simulink model "ACC_SWC"  (R2022b)
settings: configuration reference "ACC_AutosarConfig" (kept outside this file)
model workspace (MATLAB code in the model file):
  | cmdLim = Simulink.Parameter;
  | cmdLim.Value = 15;
  | cmdLim.Description = 'Limit for controlling the maximum surface command angle.';
  | cmdLim.Min = 0;
  | cmdLim.Max = 90;
  | cmdLim.DocUnits = 'deg';
  | 
  | dispGain = Simulink.Parameter;
  | dispGain.Value = 0.75;
  | dispGain.Description = 'Gain applied to the displacement error.';
  | dispGain.Min = 0;
  | dispGain.Max = [];
  | dispGain.DocUnits = 'deg/sec/deg';
  | 
  | dispLim = Simulink.Parameter;
  | dispLim.Value = 30;
  | dispLim.Description = 'Limit for controlling the maximum commanded angle.';
  | dispLim.Min = 0;
  | dispLim.Max = 180;
  | dispLim.DocUnits = 'deg';
  | 
  | intGain = Simulink.Parameter;
  | intGain.Value = 0.5;
  | intGain.Description = 'Gain applied to the integral error.';
  | intGain.Min = 0;
  | intGain.Max = [];
  | intGain.DocUnits = 'deg/sec/deg/sec';
  | 
  | intLim = Simulink.Parameter;
  | intLim.Value = 5;
  | intLim.Description = 'Limit for controlling the maximum commanded angle.';
  | intLim.Min = 0;
  | intLim.Max = 90;
  | intLim.DocUnits = 'deg';
  | 
  | rateGain = Simulink.Parameter;
  | rateGain.Value = 2;
  | rateGain.Description = 'Gain applied to the rate error.';
  | rateGain.Min = 0;
  | rateGain.Max = [];
  | rateGain.DocUnits = 'deg/deg/sec';
  | 
  | rateLim = Simulink.Parameter;
  | rateLim.Value = 6;
  | rateLim.Description = 'Limit for controlling the maximum commanded angle.';
  | rateLim.Min = 0;
  | rateLim.Max = 180;
  | rateLim.DocUnits = 'deg/sec';
  | 
  | hdgGain = Simulink.Parameter;
  | hdgGain.Value = 0.015;
values from neighbouring files (symbols this model uses):
  ACC_SampleTime = 0.01    [ACC_DD.sldd]
  Dem_EventStatusType : value not decoded    [ACC_DD.sldd]
libraries: autosarlibnvm x3, autosarlibdem x1
settings Model: RequirementInfo={} %GIDa_fe9045fd_0412_4b6e_8206_617cc20e6fde  DataDictionary=ACC_DD.sldd  FPTRunName=Active  Creator=MAAM  LastModifiedBy=MAAM
settings ConfigSetRef: SourceName=ACC_AutosarConfig

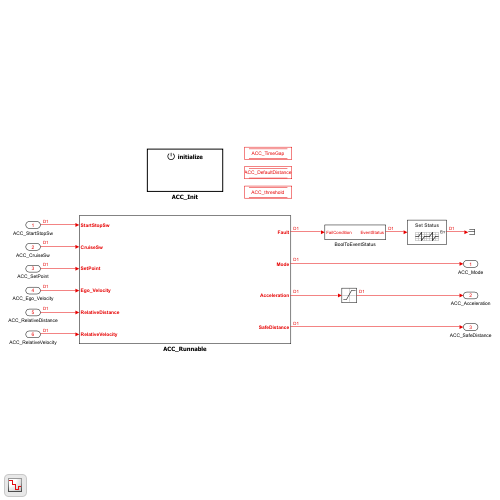
[thumbnail: Simulink's stored preview of the top-level diagram]
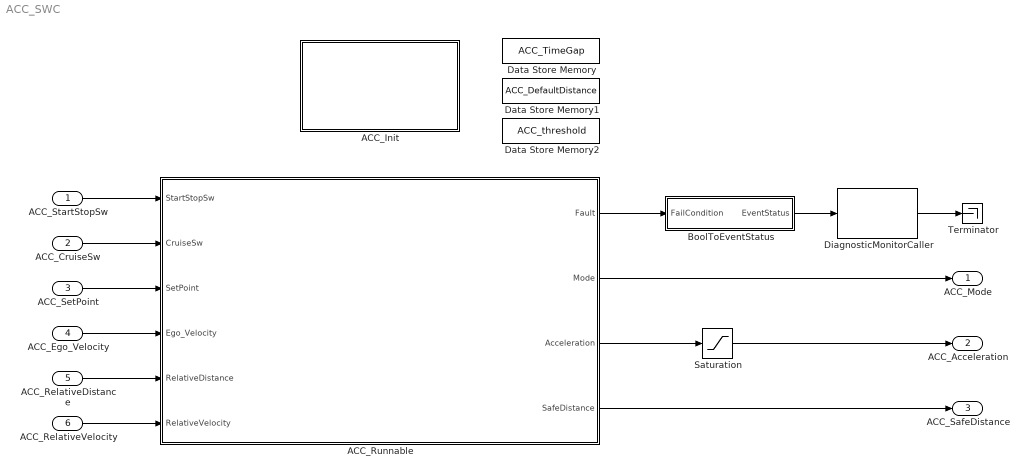
== system ACC_SWC ==
  ACC_StartStopSw : Inport  OutDataTypeStr=boolean  SampleTime=ACC_SampleTime
  ACC_CruiseSw : Inport  Port=2  OutDataTypeStr=boolean  SampleTime=ACC_SampleTime
  ACC_SetPoint : Inport  Port=3  OutDataTypeStr=single  SampleTime=ACC_SampleTime
  ACC_Ego_Velocity : Inport  Port=4  OutDataTypeStr=single  SampleTime=ACC_SampleTime
  ACC_RelativeDistance : Inport  Port=5  OutDataTypeStr=single  SampleTime=ACC_SampleTime
  ACC_RelativeVelocity : Inport  Port=6  OutDataTypeStr=single  SampleTime=ACC_SampleTime
  ACC_Init : Subsystem  TreatAsAtomicUnit=on
  ACC_Runnable : Subsystem  SystemSampleTime=1
  BoolToEventStatus : Subsystem
  Data Store Memory : DataStoreMemory  DataStoreName=ACC_TimeGap  WriteAfterWriteMsg=warning  ShowAdditionalParam=off  OutDataTypeStr=uint8
  Data Store Memory1 : DataStoreMemory  DataStoreName=ACC_DefaultDistance  WriteAfterWriteMsg=warning  ShowAdditionalParam=off  OutDataTypeStr=uint8
  Data Store Memory2 : DataStoreMemory  DataStoreName=ACC_threshold  WriteAfterWriteMsg=warning  ShowAdditionalParam=off  OutDataTypeStr=uint8
  DiagnosticMonitorCaller : autosarlibdem/DiagnosticMonitorCaller  PortName=ACC_Fail  Operation=SetEventStatus  Datatype=Enum: Dem_EventStatusType  st=-1  ServiceImpl=autosar.bsw.DemDiagnosticMonitor
  Saturation : Saturate  UpperLimit=10  LowerLimit=-10  OutDataTypeStr=single
  Terminator : Terminator
  ACC_Mode : Outport
  ACC_Acceleration : Outport  Port=2
  ACC_SafeDistance : Outport  Port=3
  wires:
  ACC_Runnable/4(SafeDistance) -> ACC_SafeDistance/1
  ACC_Runnable/3(Acceleration) -> Saturation/1
  ACC_Runnable/2(Mode) -> ACC_Mode/1
  ACC_Runnable/1(Fault) -> BoolToEventStatus/1(FailCondition)
  ACC_RelativeVelocity/1 -> ACC_Runnable/6(RelativeVelocity)
  ACC_RelativeDistance/1 -> ACC_Runnable/5(RelativeDistance)
  ACC_Ego_Velocity/1 -> ACC_Runnable/4(Ego_Velocity)
  ACC_SetPoint/1 -> ACC_Runnable/3(SetPoint)
  ACC_CruiseSw/1 -> ACC_Runnable/2(CruiseSw)
  ACC_StartStopSw/1 -> ACC_Runnable/1(StartStopSw)
  DiagnosticMonitorCaller/1 -> Terminator/1
  BoolToEventStatus/1(EventStatus) -> DiagnosticMonitorCaller/1
  Saturation/1 -> ACC_Acceleration/1

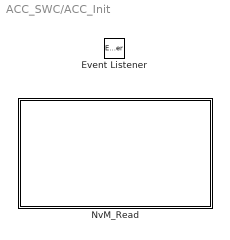
== system ACC_SWC/ACC_Init ==
  Event Listener : EventListener  DisableCoverage=on  EventName=reset
  NvM_Read : Subsystem  Tag=NvM_Read  Priority=1

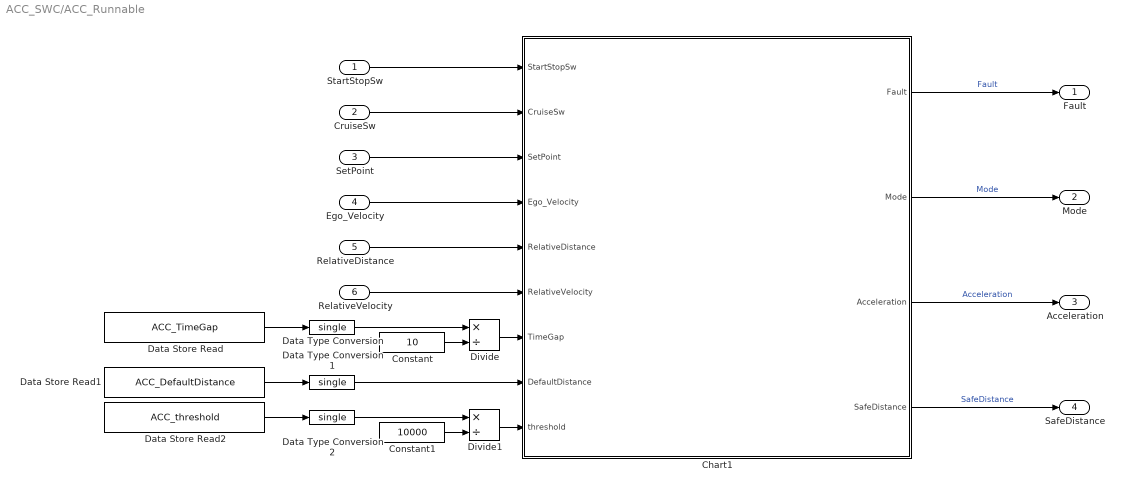
== system ACC_SWC/ACC_Runnable ==
  StartStopSw : Inport
  CruiseSw : Inport  Port=2
  SetPoint : Inport  Port=3
  Ego_Velocity : Inport  Port=4
  RelativeDistance : Inport  Port=5
  RelativeVelocity : Inport  Port=6
  Chart1 : Stateflow chart  TreatAsAtomicUnit=on
      settings: PortSchema="{\"entries\":[{\"content\":{\"sides\":[{\"content\":{\"connectorIds\":[\"In2\",\"In1\",\"In3\",\"In4\",\"In5\",\"In6\",\"In7\",\"In8\",\"In9\"]},\"type\":\"ConnectorPlacement.EquallySpacedRectSide\",\"uuid\":\"a558f2c2-5ffb-4ba0-8891-a688bb62a9b9\"},{\"content\":{\"connectorIds\":[\"Out1\",\"Out2\",\"Out3\",\"Out4\"],\"side\":\"RIGHT\"},\"type\":\"ConnectorPlacement.EquallySpacedRectSide\",\"uuid\":\"56d0d55d-a484-4316-a2b8-f7c2ba28bad9\"},{\"content\":{\"connectorIds\":[],\"side\":\"TOP\"},\"type\":\"ConnectorPlacement.EquallySpacedRectSide\",\"uuid\":\"4bb91777-42b4-417b-88ce-c76e908bf247\"}]},\"type\":\"ConnectorPlacement.EquallySpacedConnector\",\"uuid\":\"a190dafd-ffc5-4ff1-968b-a32c0c19da50\"}],\"packageUris\":[\"http://schema.mathworks.com/mf0/Connector/R2020b\"],\"version\":\"1.0\"}"
  Constant : Constant  Value=10  OutDataTypeStr=single
  Constant1 : Constant  Value=10000  OutDataTypeStr=single
  Data Store Read : DataStoreRead  DataStoreName=ACC_TimeGap  IndexOptions=Index vector (dialog)  Indices=1  OutputSizes=1
  Data Store Read1 : DataStoreRead  DataStoreName=ACC_DefaultDistance  IndexOptions=Index vector (dialog)  Indices=1  OutputSizes=1
  Data Store Read2 : DataStoreRead  DataStoreName=ACC_threshold  IndexOptions=Index vector (dialog)  Indices=1  OutputSizes=1
  Data Type Conversion : DataTypeConversion  OutDataTypeStr=single  SaturateOnIntegerOverflow=off  RndMeth=Floor
  Data Type Conversion1 : DataTypeConversion  OutDataTypeStr=single  SaturateOnIntegerOverflow=off  RndMeth=Floor
  Data Type Conversion2 : DataTypeConversion  OutDataTypeStr=single  SaturateOnIntegerOverflow=off  RndMeth=Floor
  Divide : Product  Inputs=*/  OutDataTypeStr=single
  Divide1 : Product  Inputs=*/  OutDataTypeStr=single
  Fault : Outport
  Mode : Outport  Port=2
  Acceleration : Outport  Port=3
  SafeDistance : Outport  Port=4
  wires:
  Chart1/2(Mode) -> Mode/1  "Mode"
  Chart1/3(Acceleration) -> Acceleration/1  "Acceleration"
  Chart1/4(SafeDistance) -> SafeDistance/1  "SafeDistance"
  Chart1/1(Fault) -> Fault/1  "Fault"
  Data Store Read/1 -> Data Type Conversion/1
  Data Store Read1/1 -> Data Type Conversion1/1
  Data Store Read2/1 -> Data Type Conversion2/1
  Constant/1 -> Divide/2
  Constant1/1 -> Divide1/2
  Divide/1 -> Chart1/7(TimeGap)
  Data Type Conversion/1 -> Divide/1
  Divide1/1 -> Chart1/9(threshold)
  Data Type Conversion2/1 -> Divide1/1
  StartStopSw/1 -> Chart1/2(StartStopSw)
  CruiseSw/1 -> Chart1/1(CruiseSw)
  SetPoint/1 -> Chart1/3(SetPoint)
  Ego_Velocity/1 -> Chart1/4(Ego_Velocity)
  RelativeDistance/1 -> Chart1/5(RelativeDistance)
  RelativeVelocity/1 -> Chart1/6(RelativeVelocity)
  Data Type Conversion1/1 -> Chart1/8(DefaultDistance)

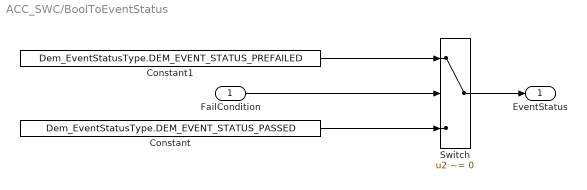
== system ACC_SWC/BoolToEventStatus ==
  FailCondition : Inport
  Constant : Constant  Value=Dem_EventStatusType.DEM_EVENT_STATUS_PASSED
  Constant1 : Constant  Value=Dem_EventStatusType.DEM_EVENT_STATUS_PREFAILED
  Switch : Switch  Criteria=u2 ~= 0  SaturateOnIntegerOverflow=off  InputSameDT=off
  EventStatus : Outport  VectorParamsAs1DForOutWhenUnconnected=off
  wires:
  Switch/1 -> EventStatus/1
  Constant1/1 -> Switch/1
  Constant/1 -> Switch/3
  FailCondition/1 -> Switch/2

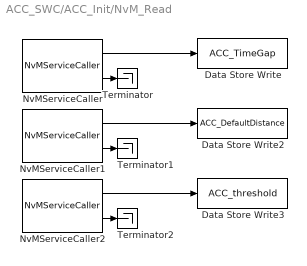
== system ACC_SWC/ACC_Init/NvM_Read ==
  Data Store Write : DataStoreWrite  DataStoreName=ACC_TimeGap  IndexOptions=Index vector (dialog)  Indices=1  OutputSizes=1
  Data Store Write2 : DataStoreWrite  DataStoreName=ACC_DefaultDistance  IndexOptions=Index vector (dialog)  Indices=1  OutputSizes=1
  Data Store Write3 : DataStoreWrite  DataStoreName=ACC_threshold  IndexOptions=Index vector (dialog)  Indices=1  OutputSizes=1
  NvMServiceCaller : autosarlibnvm/NvMServiceCaller  PortName=ACC_TimeGap_NvMService  Operation=ReadBlock  ArgumentSpecification=ACC_TimeGap_ID  st=-1  ServiceImpl=autosar.bsw.NvMService
  NvMServiceCaller1 : autosarlibnvm/NvMServiceCaller  PortName=ACC_DefaultDistance_NvMService  Operation=ReadBlock  ArgumentSpecification=ACC_DefaultDistance_ID  st=-1  ServiceImpl=autosar.bsw.NvMService
  NvMServiceCaller2 : autosarlibnvm/NvMServiceCaller  PortName=ACC_threshold_ID_NvMService  Operation=ReadBlock  ArgumentSpecification=ACC_threshold_ID  st=-1  ServiceImpl=autosar.bsw.NvMService
  Terminator : Terminator
  Terminator1 : Terminator
  Terminator2 : Terminator
  wires:
  NvMServiceCaller2/1 -> Data Store Write3/1
  NvMServiceCaller1/2 -> Terminator1/1
  NvMServiceCaller/1 -> Data Store Write/1
  NvMServiceCaller2/2 -> Terminator2/1
  NvMServiceCaller/2 -> Terminator/1
  NvMServiceCaller1/1 -> Data Store Write2/1

== stateflow chart ACC_SWC/ACC_Runnable/Chart1 ==
  state Fault_Detection_Sysytem [parallel]
    settings: executionOrder=2
    state Init
      en:
      Fault = false;
    state Wait
      en:
    state Fault
      en:
      Fault = true;
    (default) -> Init
    Init -> Wait : FaultEvent
    Wait -> Fault [order 2] : after(FaultTime, sec)
    Fault -> Fault_Detection_Sysytem : ClearEvent
    Wait -> Init [order 1] : ClearEvent
  state Regular_System [parallel]
    settings: executionOrder=1
    state CruiseControl_Activation [parallel]
      settings: executionOrder=1
      CruiseControl_Activation -> (junction 59)
      (junction 59) -> (junction 64) [order 1] : [StartStopSw && ~CruiseSw]
      (junction 59) -> (junction 62) [order 2] : {ACC_Activation = true;}
      (junction 64) -> (junction 66) : {ACC_Activation = false; Acceleration = 0; Mode = ACC_Mode.Do_Nothing;}
      (junction 66) -> (junction 62)
      (junction 62) -> CruiseControl_Activation
    state Distance_Measurement [parallel]
      en,du:
      SafeDistance = DefaultDistance + TimeGap * Ego_Velocity;
      settings: executionOrder=2
      Distance_Measurement -> (junction 83)
      (junction 83) -> (junction 85) [order 1] : [RelativeDistance >= SafeDistance]
      (junction 83) -> (junction 89) [order 2] : {send(FaultEvent, Fault_Detection_Sysytem)}
      (junction 85) -> (junction 94) : {send(ClearEvent, Fault_Detection_Sysytem)}
      (junction 94) -> (junction 89)
      (junction 89) -> Distance_Measurement
    state CruiseControl_Operation [parallel]
      settings: executionOrder=3
      CruiseControl_Operation -> (junction 151)
      (junction 151) -> (junction 71) [order 1] : [ACC_Activation]
      (junction 71) -> (junction 105) [order 1] : [(RelativeDistance - SafeDistance) >= DefaultDistance]
      (junction 105) -> (junction 99) [order 1] : [abs(SetPoint - Ego_Velocity) <= threshold]
      (junction 151) -> CruiseControl_Operation [order 2] : {Mode = ACC_Mode.Stop;}
      (junction 71) -> (junction 138) [order 2]
      (junction 105) -> (junction 108) [order 2]
      (junction 99) -> (junction 103) : {Mode = ACC_Mode.Do_Nothing;}
      (junction 108) -> (junction 110) [order 1] : [SetPoint > Ego_Velocity]
      (junction 138) -> (junction 120) : {Mode = ACC_Mode.Decelerate;}
      (junction 108) -> (junction 141) [order 2] : {Mode = ACC_Mode.Decelerate;}
      (junction 110) -> (junction 112) : {Mode = ACC_Mode.Accelerate;}
      (junction 141) -> (junction 112)
      (junction 120) -> CruiseControl_Operation : {Acceleration = ((RelativeVelocity + RelativeDistance) - SafeDistance - DefaultDistance) * 0.1;}
      (junction 112) -> CruiseControl_Operation : {Acceleration = (SetPoint - Ego_Velocity);}
      (junction 103) -> CruiseControl_Operation : {Acceleration = 0;}
  data: CruiseSw input boolean size=1; StartStopSw input boolean size=1; SetPoint input single size=1; Ego_Velocity input single size=1; RelativeDistance input single size=1; Fault output boolean size=1; Mode output size=1; FaultTime constant single =4; RelativeVelocity input single size=1; Acceleration output single size=1; SafeDistance output single size=1; ACC_Activation local; TimeGap input single =1.4; DefaultDistance input single =10; threshold input single =0.0001
  events: FaultEvent local FUNCTION_CALL_EVENT; ClearEvent local FUNCTION_CALL_EVENT
